simulink model "point_cloud_filter_transform_node"  (R2021b)
settings: Solver=FixedStepAuto  StartTime=0.0  StopTime=inf  RelTol=1e-3
model workspace (MAT data in the model file):
  Logfile_Data_Object = ros2bag
  Logfile_Data_Object.FilePath = 'C:\azumiken\lidars_point_raw\lidars_point_raw_0.db3'
  Logfile_Data_Object.StartTime = 1633675920681641206
  Logfile_Data_Object.EndTime = 1633676017682751873
  Logfile_Data_Object.AvailableTopics = table
  Logfile_Data_Object.AvailableTopics.data{1} = [969; 970]
  Logfile_Data_Object.AvailableTopics.data{2} = categorical
  Logfile_Data_Object.AvailableTopics.data{2}.categoryNames = {'sensor_msgs/PointCloud2'}
  Logfile_Data_Object.AvailableTopics.data{2}.codes = [1; 1]
  Logfile_Data_Object.AvailableTopics.data{3}{1} = '% contain additional information such as normals, intensity, etc. The
    | % point data is stored as a binary blob, its layout described by the
    | % contents of the "fields" array.
    | %
    | % The point cloud data may be organized 2d (image-like) or 1d (unordered).
    | % Point clouds organized as 2d images may be produced by camera depth sensors
    | % such as stereo or Time-of-flight.
    | 
    | % Time of sensor data acquisition, and the coordinate frame ID (for 3d points).
    | std_msgs/Header header
    | 
    | % 2D structure of the point cloud. If the cloud is unordered, height is
    | % 1 and width is the length of the point cloud.
    | uint32 height
    | uint32 width
    | 
    | % Describes the channels and their layout in the binary data blob.
    | PointField[] fields
    | 
    | logical    is_bigendian % Is this data bigendian?
    | uint32  point_step      % Length of a point in bytes
    | uint32  row_step        % Length of a row in bytes
    | uint8[] data            % Actual point data, size is (row_step*height)
    | 
    | logical is_dense        % True if there are no invalid points'
  Logfile_Data_Object.AvailableTopics.data{3}{2} = '% contain additional information such as normals, intensity, etc. The
    | % point data is stored as a binary blob, its layout described by the
    | % contents of the "fields" array.
    | %
    | % The point cloud data may be organized 2d (image-like) or 1d (unordered).
    | % Point clouds organized as 2d images may be produced by camera depth sensors
    | % such as stereo or Time-of-flight.
    | 
    | % Time of sensor data acquisition, and the coordinate frame ID (for 3d points).
    | std_msgs/Header header
    | 
    | % 2D structure of the point cloud. If the cloud is unordered, height is
    | % 1 and width is the length of the point cloud.
    | uint32 height
    | uint32 width
    | 
    | % Describes the channels and their layout in the binary data blob.
    | PointField[] fields
    | 
    | logical    is_bigendian % Is this data bigendian?
    | uint32  point_step      % Length of a point in bytes
    | uint32  row_step        % Length of a row in bytes
    | uint8[] data            % Actual point data, size is (row_step*height)
    | 
    | logical is_dense        % True if there are no invalid points'
  Logfile_Data_Object.AvailableTopics.ndims = 2
  Logfile_Data_Object.AvailableTopics.nrows = 2
  Logfile_Data_Object.AvailableTopics.rownames = {'/lidar_front/points_raw'; '/lidar_rear/points_raw'}
  Logfile_Data_Object.AvailableTopics.nvars = 3
  Logfile_Data_Object.AvailableTopics.varnames = {'NumMessages', 'MessageType', 'MessageDefinition'}
  Logfile_Data_Object.AvailableTopics.props.useVariableNamesOriginal = 0
  Logfile_Data_Object.AvailableTopics.props.useDimensionNamesOriginal = 0
  Logfile_Data_Object.AvailableTopics.props.CustomProps = struct()
  Logfile_Data_Object.AvailableTopics.props.VariableCustomProps = struct()
  Logfile_Data_Object.AvailableTopics.props.versionSavedFrom = 4
  Logfile_Data_Object.AvailableTopics.props.minCompatibleVersion = 1
  Logfile_Data_Object.AvailableTopics.props.incompatibilityMsg = ''
  Logfile_Data_Object.AvailableTopics.props.VersionSavedFrom = 4
  Logfile_Data_Object.AvailableTopics.props.Description = ''
  Logfile_Data_Object.AvailableTopics.props.VariableNamesOriginal = {}
  Logfile_Data_Object.AvailableTopics.props.DimensionNames = {'Row', 'Variables'}
  Logfile_Data_Object.AvailableTopics.props.DimensionNamesOriginal = {}
  Logfile_Data_Object.AvailableTopics.props.UserData = []
  Logfile_Data_Object.AvailableTopics.props.VariableDescriptions = {}
  Logfile_Data_Object.AvailableTopics.props.VariableUnits = {}
  Logfile_Data_Object.AvailableTopics.props.VariableContinuity = {}
  Logfile_Data_Object.MessageList = table
  Logfile_Data_Object.MessageList.data{1} = [1633675920681641206 1633675920704850047 1633675920710280571 1633675920841302537 1633675920849007917 1633675920944718285 1633675920950454411 1633675921046456357 1633675921051238695 1633675921143527086 1633675921154682295 1633675921262758351 ... (1939 elements, 1939x1)]
  Logfile_Data_Object.MessageList.data{2} = categorical
  Logfile_Data_Object.MessageList.data{2}.categoryNames = {'/lidar_rear/points_raw'; '/lidar_front/points_raw'}
  Logfile_Data_Object.MessageList.data{2}.codes = [1 2 1 2 1 2 1 2 1 2 1 2 ... (1939 elements, 1939x1)]
  Logfile_Data_Object.MessageList.data{3} = categorical
  Logfile_Data_Object.MessageList.data{3}.categoryNames = {'sensor_msgs/PointCloud2'}
  Logfile_Data_Object.MessageList.data{3}.codes = [1 1 1 1 1 1 1 1 1 1 1 1 ... (1939 elements, 1939x1)]
  Logfile_Data_Object.MessageList.ndims = 2
  Logfile_Data_Object.MessageList.nrows = 1939
  Logfile_Data_Object.MessageList.nvars = 3
  Logfile_Data_Object.MessageList.varnames = {'Time', 'Topic', 'MessageType'}
  Logfile_Data_Object.MessageList.props.useVariableNamesOriginal = 0
  Logfile_Data_Object.MessageList.props.useDimensionNamesOriginal = 0
  Logfile_Data_Object.MessageList.props.CustomProps = struct()
  Logfile_Data_Object.MessageList.props.VariableCustomProps = struct()
  Logfile_Data_Object.MessageList.props.versionSavedFrom = 4
  Logfile_Data_Object.MessageList.props.minCompatibleVersion = 1
  Logfile_Data_Object.MessageList.props.incompatibilityMsg = ''
  Logfile_Data_Object.MessageList.props.VersionSavedFrom = 4
  Logfile_Data_Object.MessageList.props.Description = ''
  Logfile_Data_Object.MessageList.props.VariableNamesOriginal = {}
  Logfile_Data_Object.MessageList.props.DimensionNames = {'Row', 'Variables'}
  Logfile_Data_Object.MessageList.props.DimensionNamesOriginal = {}
  Logfile_Data_Object.MessageList.props.UserData = []
  Logfile_Data_Object.MessageList.props.VariableDescriptions = {}
  Logfile_Data_Object.MessageList.props.VariableUnits = {}
  Logfile_Data_Object.MessageList.props.VariableContinuity = {}
  Logfile_Data_Object.TopicTypeMap = containers.Map
  Logfile_Data_Object.TopicTypeMap.serialization.keys = {'/lidar_front/points_raw', '/lidar_rear/points_raw'}
  Logfile_Data_Object.TopicTypeMap.serialization.values = {'sensor_msgs/PointCloud2', 'sensor_msgs/PointCloud2'}
  Logfile_Data_Object.TopicTypeMap.serialization.uniformity = 1
  Logfile_Data_Object.TopicTypeMap.serialization.keyType = 'char'
  Logfile_Data_Object.TopicTypeMap.serialization.valueType = 'char'
  Logfile_Data_Object.TopicDefinitionMap = containers.Map
  Logfile_Data_Object.TopicDefinitionMap.serialization.keys = {'/lidar_front/points_raw', '/lidar_rear/points_raw'}
  Logfile_Data_Object.TopicDefinitionMap.serialization.values{1} = '% contain additional information such as normals, intensity, etc. The
    | % point data is stored as a binary blob, its layout described by the
    | % contents of the "fields" array.
    | %
    | % The point cloud data may be organized 2d (image-like) or 1d (unordered).
    | % Point clouds organized as 2d images may be produced by camera depth sensors
    | % such as stereo or Time-of-flight.
    | 
    | % Time of sensor data acquisition, and the coordinate frame ID (for 3d points).
    | std_msgs/Header header
    | 
    | % 2D structure of the point cloud. If the cloud is unordered, height is
    | % 1 and width is the length of the point cloud.
    | uint32 height
    | uint32 width
    | 
    | % Describes the channels and their layout in the binary data blob.
    | PointField[] fields
    | 
    | logical    is_bigendian % Is this data bigendian?
    | uint32  point_step      % Length of a point in bytes
    | uint32  row_step        % Length of a row in bytes
    | uint8[] data            % Actual point data, size is (row_step*height)
    | 
    | logical is_dense        % True if there are no invalid points'
  Logfile_Data_Object.TopicDefinitionMap.serialization.values{2} = '% contain additional information such as normals, intensity, etc. The
    | % point data is stored as a binary blob, its layout described by the
    | % contents of the "fields" array.
    | %
    | % The point cloud data may be organized 2d (image-like) or 1d (unordered).
    | % Point clouds organized as 2d images may be produced by camera depth sensors
    | % such as stereo or Time-of-flight.
    | 
    | % Time of sensor data acquisition, and the coordinate frame ID (for 3d points).
    | std_msgs/Header header
    | 
    | % 2D structure of the point cloud. If the cloud is unordered, height is
    | % 1 and width is the length of the point cloud.
    | uint32 height
    | uint32 width
    | 
    | % Describes the channels and their layout in the binary data blob.
    | PointField[] fields
    | 
    | logical    is_bigendian % Is this data bigendian?
    | uint32  point_step      % Length of a point in bytes
    | uint32  row_step        % Length of a row in bytes
    | uint8[] data            % Actual point data, size is (row_step*height)
    | 
    | logical is_dense        % True if there are no invalid points'
  Logfile_Data_Object.TopicDefinitionMap.serialization.uniformity = 1
  Logfile_Data_Object.TopicDefinitionMap.serialization.keyType = 'char'
  Logfile_Data_Object.TopicDefinitionMap.serialization.valueType = 'char'
  Logfile_Path = 'C:\azumiken\lidars_point_raw\lidars_point_raw_0.db3'
  Logfile_Playback_Duration = nan
  Logfile_Playback_Offset = nan
  SL_ROS_VariableLengthArrays_MaxSizes.CommonInfo.ArrayTruncateAction = 'EmitWarning'
  SL_ROS_VariableLengthArrays_MaxSizes.MsgTypeMap = containers.Map
  SL_ROS_VariableLengthArrays_MaxSizes.MsgTypeMap.serialization.keys = {'sensor_msgs/PointCloud2'}
  SL_ROS_VariableLengthArrays_MaxSizes.MsgTypeMap.serialization.values{1}(1).PropertyName = 'data'
  SL_ROS_VariableLengthArrays_MaxSizes.MsgTypeMap.serialization.values{1}(1).DataType = 'uint8'
  SL_ROS_VariableLengthArrays_MaxSizes.MsgTypeMap.serialization.values{1}(1).MaxLength = 220000
  SL_ROS_VariableLengthArrays_MaxSizes.MsgTypeMap.serialization.values{1}(2).PropertyName = 'fields'
  SL_ROS_VariableLengthArrays_MaxSizes.MsgTypeMap.serialization.values{1}(2).DataType = 'sensor_msgs/PointField'
  SL_ROS_VariableLengthArrays_MaxSizes.MsgTypeMap.serialization.values{1}(2).MaxLength = 16
  SL_ROS_VariableLengthArrays_MaxSizes.MsgTypeMap.serialization.uniformity = 0
  SL_ROS_VariableLengthArrays_MaxSizes.MsgTypeMap.serialization.keyType = 'char'
  SL_ROS_VariableLengthArrays_MaxSizes.MsgTypeMap.serialization.valueType = 'any'
undefined symbols (not defined in the file or in its folder): height, row_step, width
libraries: ros2lib x4, simulink x4
settings Model: Creator=takum  LastModifiedBy=takumi onozawa
settings OptimizationCC: DefaultParameterBehavior=Inlined  EnhancedBackFolding=on  PassReuseOutputArgsAs=Individual arguments  ZeroExternalMemoryAtStartup=off  ZeroInternalMemoryAtStartup=off  MaxStackSize=64  OptimizeBlockOrder=speed  DifferentSizesBufferReuse=on  OptimizationCustomize=off  EfficientTunableParamExpr=on
settings DebuggingCC: ParameterTunabilityLossMsg=error
settings SFSimCC: SimParseCustomCode=off  SimTargetLang=C++
settings RTWCC: Description=Embedded Coder  SystemTargetFile=ert.tlc  HardwareBoard=Robot Operating System 2 (ROS 2)  TemplateMakefile=ert_default_tmf  Toolchain=Colcon Tools
settings CodeAppCC: ForceParamTrailComments=on  IgnoreCustomStorageClasses=off  OperatorAnnotations=on  SimulinkDataObjDesc=on  SFDataObjDesc=on  InsertBlockDesc=on
settings ERTTargetCC: TargetLangStandard=C99 (ISO)  InlinedParameterPlacement=NonHierarchical  ERTCustomFileTemplate=example_file_process.tlc

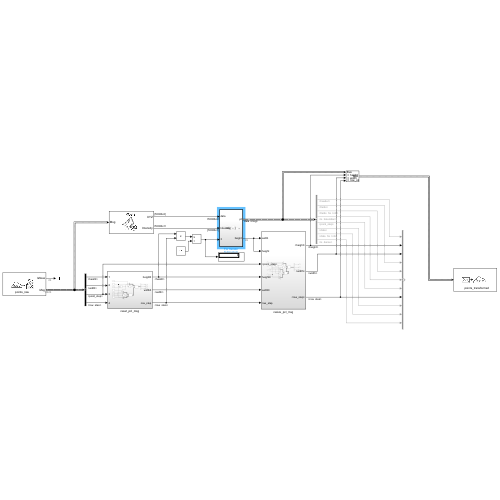
[thumbnail: Simulink's stored preview of the top-level diagram]
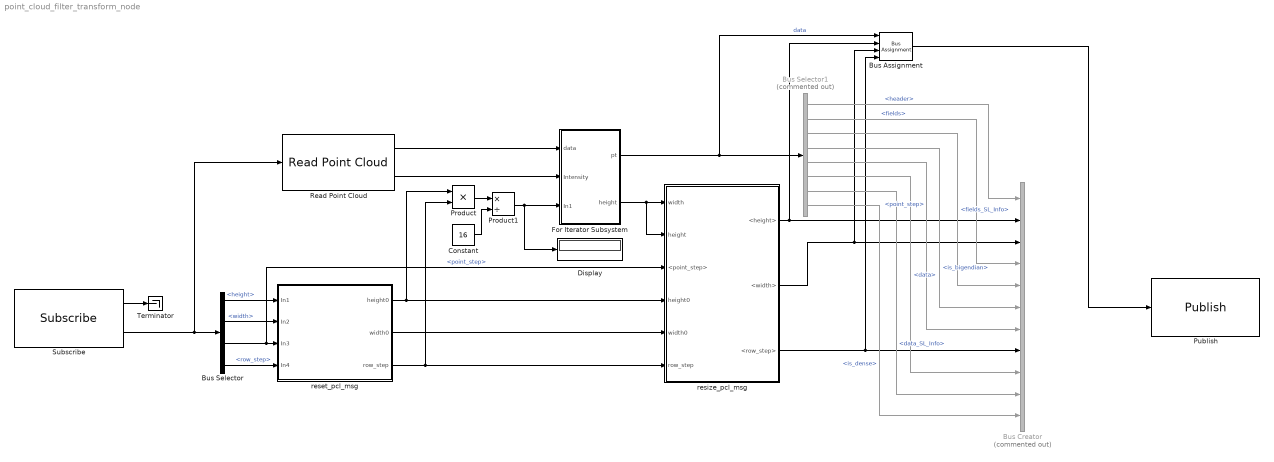
== system point_cloud_filter_transform_node ==
  Bus Assignment : BusAssignment  AssignedSignals=height,width,row_step
  Bus Creator : BusCreator  Commented=on  Inputs=11
  Bus Selector : BusSelector  OutputSignals=height,width,point_step,row_step
  Bus Selector1 : BusSelector  Commented=on  OutputSignals=header,fields,fields_SL_Info,is_bigendian,point_step,data,data_SL_Info,is_dense
  Constant : Constant  Value=16  OutDataTypeStr=uint32
  Display : Display
  For Iterator Subsystem : Subsystem  TreatAsAtomicUnit=on
  Product : Product  OutDataTypeStr=uint32
  Product1 : Product  Inputs=*/  OutDataTypeStr=uint32
  Publish : ros2lib/Publish  topicSource=Specify your own  topic=points_transformed  messageType=sensor_msgs/PointCloud2  QOSHistory=Keep last  QOSDepth=1  QOSReliability=Reliable  QOSDurability=Volatile
      settings: SourceProductBaseCode=RR
  Read Point Cloud : ros2lib/Read Point Cloud  MaximumPointCloudSize=[1, 55000]  PreserveStructure=off  ShowRGBOutput=off  ShowIntensityOutput=on  ShowErrorCodeOutput=off  VariableSizeOutputs=off
      settings: SourceProductBaseCode=RR
  Subscribe : ros2lib/Subscribe  topicSource=Specify your own  topic=points_raw  messageType=sensor_msgs/PointCloud2  sampleTime=-1  QOSHistory=Keep last  QOSDepth=1  QOSReliability=Reliable  QOSDurability=Volatile
      settings: SourceProductBaseCode=RR
  Terminator : Terminator
  reset_pcl_msg : Subsystem
  resize_pcl_msg : Subsystem
  wires:
  Subscribe/1 -> Terminator/1
  Bus Assignment/1 -> Publish/1
  resize_pcl_msg/1(<height>) -> Bus Assignment/2, Bus Creator/2
  Subscribe/2 -> Bus Selector/1, Read Point Cloud/1
  Bus Selector/2 -> reset_pcl_msg/2(In2)  "<width>"
  reset_pcl_msg/1(height0) -> resize_pcl_msg/4(height0), Product/1
  Product/1 -> Product1/1
  Bus Selector/4 -> reset_pcl_msg/4(In4)  "<row_step>"
  Product1/1 -> Display/1, For Iterator Subsystem/3(In1)
  For Iterator Subsystem/2(height) -> resize_pcl_msg/2(height), resize_pcl_msg/1(width)
  reset_pcl_msg/2(width0) -> resize_pcl_msg/5(width0)
  Constant/1 -> Product1/2
  reset_pcl_msg/3(row_step) -> resize_pcl_msg/6(row_step), Product/2
  Bus Selector/1 -> reset_pcl_msg/1(In1)  "<height>"
  Bus Selector/3 -> resize_pcl_msg/3(<point_step>), reset_pcl_msg/3(In3)  "<point_step>"
  resize_pcl_msg/3(<row_step>) -> Bus Assignment/4, Bus Creator/8
  resize_pcl_msg/2(<width>) -> Bus Assignment/3, Bus Creator/3
  Read Point Cloud/1 -> For Iterator Subsystem/1(data)
  Read Point Cloud/2 -> For Iterator Subsystem/2(Intensity)
  For Iterator Subsystem/1(pt) -> Bus Assignment/1, Bus Selector1/1  "data"
  Bus Selector1/1 -> Bus Creator/1  "<header>"
  Bus Selector1/2 -> Bus Creator/4  "<fields>"
  Bus Selector1/3 -> Bus Creator/5  "<fields_SL_Info>"
  Bus Selector1/4 -> Bus Creator/6  "<is_bigendian>"
  Bus Selector1/5 -> Bus Creator/7  "<point_step>"
  Bus Selector1/6 -> Bus Creator/9  "<data>"
  Bus Selector1/7 -> Bus Creator/10  "<data_SL_Info>"
  Bus Selector1/8 -> Bus Creator/11  "<is_dense>"

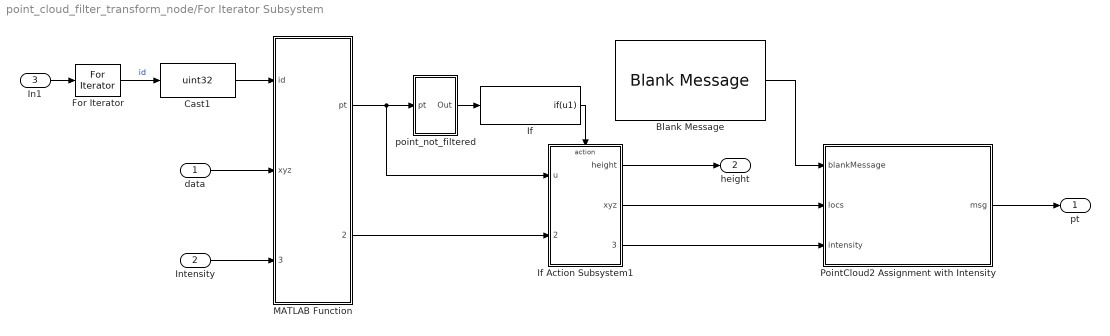
== system point_cloud_filter_transform_node/For Iterator Subsystem ==
  data : Inport
  Intensity : Inport  Port=2
  In1 : Inport  Port=3
  Blank Message : ros2lib/Blank Message  messageClass=Message  entityType=sensor_msgs/PointCloud2  messageType=sensor_msgs/PointCloud2  SampleTime=inf
      settings: SourceProductBaseCode=RR
  Cast1 : DataTypeConversion  OutDataTypeStr=uint32
  For Iterator : ForIterator  IterationSource=external
  If : If  IfExpression=u1  ShowElse=off
  If Action Subsystem1 : Subsystem  TreatAsAtomicUnit=on
  MATLAB Function : MATLAB Function  TreatAsAtomicUnit=on
  PointCloud2 Assignment with Intensity : MATLAB Function  TreatAsAtomicUnit=on
  point_not_filtered : Subsystem
  pt : Outport
  height : Outport  Port=2
  wires:
  If Action Subsystem1/2(xyz) -> PointCloud2 Assignment with Intensity/2(locs)
  If Action Subsystem1/3(intensity) -> PointCloud2 Assignment with Intensity/3(intensity)
  If Action Subsystem1/1(height) -> height/1
  Cast1/1 -> MATLAB Function/1(id)
  PointCloud2 Assignment with Intensity/1(msg) -> pt/1
  Intensity/1 -> MATLAB Function/3(Intensity)
  For Iterator/1 -> Cast1/1  "id"
  data/1 -> MATLAB Function/2(xyz)
  MATLAB Function/1(pt) -> If Action Subsystem1/1(u), point_not_filtered/1(pt)
  point_not_filtered/1(Out) -> If/1
  In1/1 -> For Iterator/1
  Blank Message/1 -> PointCloud2 Assignment with Intensity/1(blankMessage)
  MATLAB Function/2(intensity) -> If Action Subsystem1/2(Intensity)
  If/1 -> If Action Subsystem1/Action

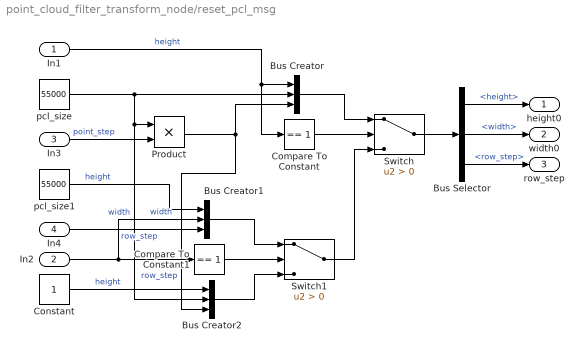
== system point_cloud_filter_transform_node/reset_pcl_msg ==
  In1 : Inport
  In2 : Inport  Port=2
  In3 : Inport  Port=3
  In4 : Inport  Port=4
  Bus Creator : BusCreator  Inputs=3
  Bus Creator1 : BusCreator  Inputs=3
  Bus Creator2 : BusCreator  Inputs=3
  Bus Selector : BusSelector  OutputSignals=height,width,row_step
  Compare To Constant : simulink/Logic and Bit Operations/Compare To Constant  relop===  const=1  OutDataTypeStr=boolean
  Compare To Constant1 : simulink/Logic and Bit Operations/Compare To Constant  relop===  const=1  OutDataTypeStr=boolean
  Constant : Constant  OutDataTypeStr=uint32
  Product : Product  OutDataTypeStr=uint32
  Switch : Switch  Criteria=u2 > Threshold
  Switch1 : Switch  Criteria=u2 > Threshold
  pcl_size : Constant  Value=55000  OutDataTypeStr=uint32
  pcl_size1 : Constant  Value=55000  OutDataTypeStr=uint32
  height0 : Outport
  width0 : Outport  Port=2
  row_step : Outport  Port=3
  wires:
  In3/1 -> Product/2  "point_step"
  In1/1 -> Compare To Constant/1, Bus Creator/1  "height"
  Compare To Constant/1 -> Switch/2
  Bus Creator/1 -> Switch/1
  Compare To Constant1/1 -> Switch1/2
  pcl_size1/1 -> Bus Creator1/1  "height"
  Bus Creator1/1 -> Switch1/1
  In2/1 -> Bus Creator1/2, Compare To Constant1/1  "width"
  In4/1 -> Bus Creator1/3  "row_step"
  Switch1/1 -> Switch/3
  Product/1 -> Bus Creator2/3, Bus Creator/3  "row_step"
  pcl_size/1 -> Bus Creator/2, Bus Creator2/2, Product/1  "width"
  Constant/1 -> Bus Creator2/1  "height"
  Bus Creator2/1 -> Switch1/3
  Switch/1 -> Bus Selector/1
  Bus Selector/2 -> width0/1  "<width>"
  Bus Selector/1 -> height0/1  "<height>"
  Bus Selector/3 -> row_step/1  "<row_step>"

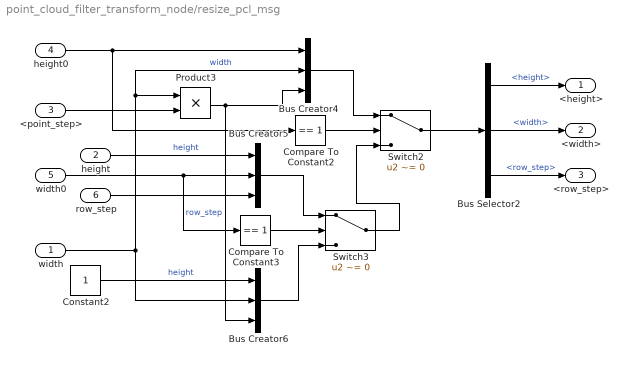
== system point_cloud_filter_transform_node/resize_pcl_msg ==
  width : Inport
  height : Inport  Port=2
  <point_step> : Inport  Port=3
  height0 : Inport  Port=4
  width0 : Inport  Port=5
  row_step : Inport  Port=6
  Bus Creator4 : BusCreator  Inputs=3
  Bus Creator5 : BusCreator  Inputs=3
  Bus Creator6 : BusCreator  Inputs=3
  Bus Selector2 : BusSelector  OutputSignals=height,width,row_step
  Compare To Constant2 : simulink/Logic and Bit Operations/Compare To Constant  relop===  const=1  OutDataTypeStr=boolean
  Compare To Constant3 : simulink/Logic and Bit Operations/Compare To Constant  relop===  const=1  OutDataTypeStr=boolean
  Constant2 : Constant  OutDataTypeStr=uint32
  Product3 : Product  OutDataTypeStr=uint32
  Switch2 : Switch  Criteria=u2 ~= 0
  Switch3 : Switch  Criteria=u2 ~= 0
  <height> : Outport
  <width> : Outport  Port=2
  <row_step> : Outport  Port=3
  wires:
  Compare To Constant3/1 -> Switch3/2
  Bus Creator6/1 -> Switch3/3
  Switch2/1 -> Bus Selector2/1
  Product3/1 -> Bus Creator4/3, Bus Creator6/3  "row_step"
  Switch3/1 -> Switch2/3
  Bus Selector2/1 -> <height>/1  "<height>"
  width/1 -> Bus Creator6/2, Bus Creator4/2, Product3/1  "width"
  Bus Creator5/1 -> Switch3/1
  Constant2/1 -> Bus Creator6/1  "height"
  Bus Creator4/1 -> Switch2/1
  Compare To Constant2/1 -> Switch2/2
  height0/1 -> Compare To Constant2/1, Bus Creator4/1
  width0/1 -> Compare To Constant3/1, Bus Creator5/2
  Bus Selector2/3 -> <row_step>/1  "<row_step>"
  <point_step>/1 -> Product3/2
  row_step/1 -> Bus Creator5/3
  Bus Selector2/2 -> <width>/1  "<width>"
  height/1 -> Bus Creator5/1  "height"

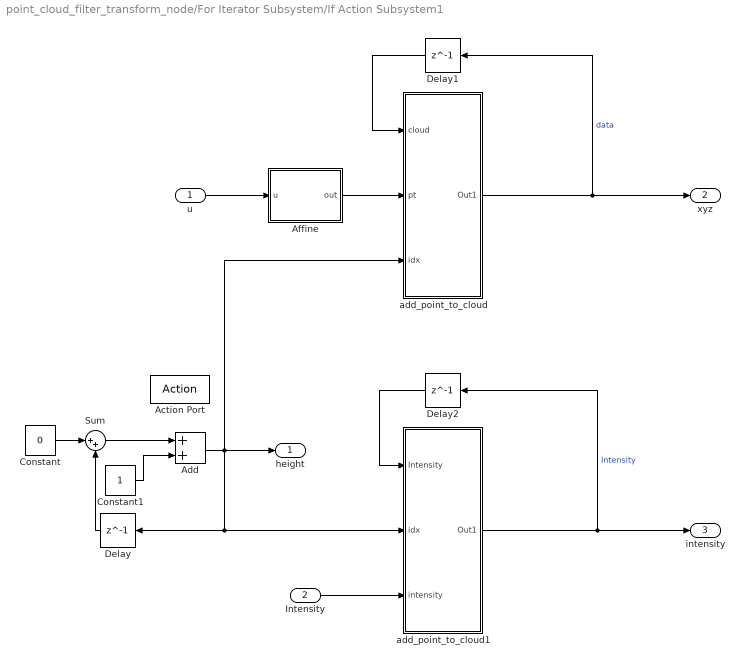
== system point_cloud_filter_transform_node/For Iterator Subsystem/If Action Subsystem1 ==
  u : Inport
  Intensity : Inport  Port=2
  Action Port : ActionPort  ActionPortLabel=if(u1)
  Add : Sum
  Affine : MATLAB Function  TreatAsAtomicUnit=on
  Constant : Constant  Value=0
  Constant1 : Constant
  Delay : Delay  DelayLength=1
  Delay1 : Delay  DelayLength=1  InitialCondition=0
  Delay2 : Delay  DelayLength=1  InitialCondition=0
  Sum : Sum  Inputs=|++
  add_point_to_cloud : Subsystem
  add_point_to_cloud1 : Subsystem
  height : Outport
  xyz : Outport  Port=2
  intensity : Outport  Port=3
  wires:
  u/1 -> Affine/1(u)
  Delay1/1 -> add_point_to_cloud/1(cloud)
  Add/1 -> add_point_to_cloud/3(idx), Delay/1, add_point_to_cloud1/2(idx), height/1
  Constant1/1 -> Add/2
  Sum/1 -> Add/1
  Constant/1 -> Sum/1
  Delay/1 -> Sum/2
  add_point_to_cloud/1(Out1) -> xyz/1, Delay1/1  "data"
  Affine/1(out) -> add_point_to_cloud/2(pt)
  Intensity/1 -> add_point_to_cloud1/3(intensity)
  Delay2/1 -> add_point_to_cloud1/1(Intensity)
  add_point_to_cloud1/1(Out1) -> Delay2/1, intensity/1  "Intensity"

== system point_cloud_filter_transform_node/For Iterator Subsystem/point_not_filtered ==
  pt : Inport
  Logical Operator2 : Logic  AllPortsSameDT=off  OutDataTypeStr=boolean
  m_angle_filter : Subsystem
  m_distance_filter : Subsystem
  Out : Outport
  wires:
  pt/1 -> m_angle_filter/1(pt), m_distance_filter/1(pt)
  Logical Operator2/1 -> Out/1
  m_distance_filter/1(Out1) -> Logical Operator2/2
  m_angle_filter/1(Out1) -> Logical Operator2/1

== system point_cloud_filter_transform_node/For Iterator Subsystem/If Action Subsystem1/add_point_to_cloud ==
  cloud : Inport
  pt : Inport  Port=2
  idx : Inport  Port=3
  MATLAB Function : MATLAB Function  TreatAsAtomicUnit=on
  MATLAB Function1 : MATLAB Function  TreatAsAtomicUnit=on
  Switch : Switch  Criteria=u2 ~= 0
  Out1 : Outport
  wires:
  MATLAB Function/1(cloud) -> Switch/1
  cloud/1 -> Switch/2, MATLAB Function/1("cloud ")
  pt/1 -> MATLAB Function1/1(pt), MATLAB Function/2(pt)
  idx/1 -> MATLAB Function/3(idx)
  Switch/1 -> Out1/1
  MATLAB Function1/1(cloud) -> Switch/3

== system point_cloud_filter_transform_node/For Iterator Subsystem/If Action Subsystem1/add_point_to_cloud1 ==
  Intensity : Inport
  idx : Inport  Port=2
  intensity : Inport  Port=3
  MATLAB Function : MATLAB Function  TreatAsAtomicUnit=on
  MATLAB Function2 : MATLAB Function  TreatAsAtomicUnit=on
  Switch : Switch  Criteria=u2 ~= 0
  Out1 : Outport
  wires:
  idx/1 -> MATLAB Function/2(j)
  intensity/1 -> MATLAB Function2/1(intensity), MATLAB Function/3(intensity)
  Intensity/1 -> MATLAB Function/1("Intensity "), Switch/2
  MATLAB Function2/1(Intensity) -> Switch/3
  MATLAB Function/1(Intensity) -> Switch/1
  Switch/1 -> Out1/1

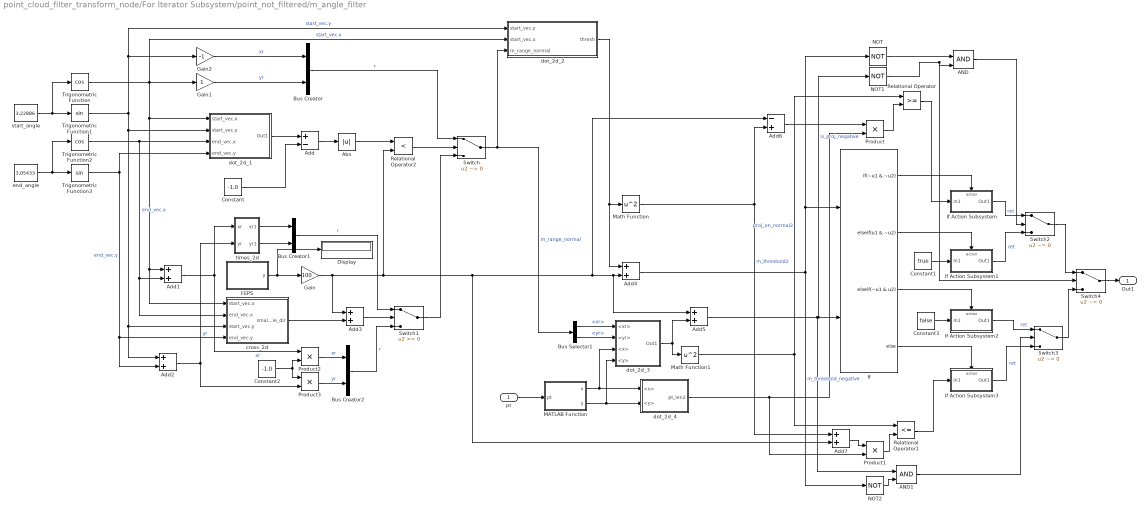
== system point_cloud_filter_transform_node/For Iterator Subsystem/point_not_filtered/m_angle_filter ==
  pt : Inport
  AND : Logic  IconShape=distinctive  AllPortsSameDT=off  OutDataTypeStr=boolean
  AND1 : Logic  IconShape=distinctive  AllPortsSameDT=off  OutDataTypeStr=boolean
  Abs : Abs
  Add : Sum  Inputs=+-
  Add{1..5,7} (6 alike) : Sum
  Add6 : Sum  Inputs=-+
  Bus Creator : BusCreator  Inputs=2
  Bus Creator1 : BusCreator  Inputs=2
  Bus Creator2 : BusCreator  Inputs=2
  Bus Selector1 : BusSelector  OutputSignals=xr,yr
  Constant : Constant  Value=-1.0
  Constant1 : Constant  Value=true  OutDataTypeStr=boolean
  Constant2 : Constant  Value=-1.0
  Constant3 : Constant  Value=false  OutDataTypeStr=boolean
  Display : Display
  FEPS : MATLAB Function  TreatAsAtomicUnit=on
  Gain : Gain  Gain=100
  Gain1 : Gain
  Gain2 : Gain  Gain=-1
  If : If  NumInputs=2  IfExpression=~u1 & ~u2  ElseIfExpressions=u1 & ~u2, ~u1 & u2
  If Action Subsystem : Subsystem  TreatAsAtomicUnit=on
  If Action Subsystem1 : Subsystem  TreatAsAtomicUnit=on
  If Action Subsystem2 : Subsystem  TreatAsAtomicUnit=on
  If Action Subsystem3 : Subsystem  TreatAsAtomicUnit=on
  MATLAB Function : MATLAB Function  TreatAsAtomicUnit=on
  Math Function : Math  Operator=square  SaturateOnIntegerOverflow=on
  Math Function1 : Math  Operator=square  SaturateOnIntegerOverflow=on
  NOT : Logic  Operator=NOT  IconShape=distinctive  AllPortsSameDT=off  OutDataTypeStr=boolean
  NOT1 : Logic  Operator=NOT  IconShape=distinctive  AllPortsSameDT=off  OutDataTypeStr=boolean
  NOT2 : Logic  Operator=NOT  IconShape=distinctive  AllPortsSameDT=off  OutDataTypeStr=boolean
  Product{,1..3} (4 alike) : Product
  Relational Operator : RelationalOperator  OutDataTypeStr=boolean  RndMeth=Simplest
  Relational Operator1 : RelationalOperator  Operator=<=  OutDataTypeStr=boolean  RndMeth=Simplest
  Relational Operator2 : RelationalOperator  Operator=<  OutDataTypeStr=boolean  RndMeth=Simplest
  Switch{,2..4} (4 alike) : Switch  Criteria=u2 ~= 0
  Switch1 : Switch
  Trigonometric Function : Trigonometry  Operator=cos
  Trigonometric Function1 : Trigonometry
  Trigonometric Function2 : Trigonometry  Operator=cos
  Trigonometric Function3 : Trigonometry
  cross_2d : Subsystem
  dot_2d_1 : Subsystem
  dot_2d_2 : Subsystem
  dot_2d_3 : Subsystem
  dot_2d_4 : Subsystem
  end_angle : Constant  Value=3.05433
  start_angle : Constant  Value=3.22886
  times_2d : Subsystem
  Out1 : Outport
  wires:
  pt/1 -> MATLAB Function/1(pt)
  start_angle/1 -> Trigonometric Function1/1, Trigonometric Function/1
  end_angle/1 -> Trigonometric Function3/1, Trigonometric Function2/1
  Trigonometric Function/1 -> dot_2d_2/2(start_vec.x), cross_2d/1(start_vec.x), Add1/1, dot_2d_1/1(start_vec.x), Gain1/1  "start_vec.x"
  Trigonometric Function1/1 -> dot_2d_1/2(start_vec.y), Add2/1, cross_2d/3(start_vec.y), dot_2d_2/1(start_vec.y), Gain2/1  "start_vec.y"
  Trigonometric Function2/1 -> cross_2d/2(end_vec.x), Add1/2, dot_2d_1/3(end_vec.x)  "end_vec.x"
  Trigonometric Function3/1 -> Add2/2, cross_2d/4(end_vec.y), dot_2d_1/4(end_vec.y)  "end_vec.y"
  dot_2d_1/1(Out1) -> Add/1
  Constant/1 -> Add/2
  Add/1 -> Abs/1
  FEPS/1(y) -> Gain/1, Display/1
  Abs/1 -> Relational Operator2/1
  Relational Operator2/1 -> Switch/2
  Gain1/1 -> Bus Creator/2  "yr"
  Gain2/1 -> Bus Creator/1  "xr"
  Bus Creator/1 -> Switch/1  "r"
  Add1/1 -> times_2d/1(xr), Product2/1  "xr"
  Add2/1 -> times_2d/2(yr), Product3/2  "yr"
  Switch1/1 -> Switch/3
  Product3/1 -> Bus Creator2/2  "yr"
  Bus Creator2/1 -> Switch1/3  "r"
  Product2/1 -> Bus Creator2/1  "xr"
  Bus Creator1/1 -> Switch1/1  "r"
  Constant2/1 -> Product2/2, Product3/1
  Add3/1 -> Switch1/2
  cross_2d/1(small_angle_dir) -> Add3/2
  times_2d/1(xr1) -> Bus Creator1/1
  times_2d/2(yr1) -> Bus Creator1/2
  Switch/1 -> Bus Selector1/1, dot_2d_2/3(m_range_normal)  "m_range_normal"
  dot_2d_2/1(thresh) -> Add4/1, Math Function/1
  Math Function/1 -> Add6/2, Add7/1  "m_threshold2"
  Add4/1 -> NOT2/1, NOT/1, If/1  "m_threshold_negative"
  Gain/1 -> Add3/1, Relational Operator2/2, Add7/2, Add6/1, Add5/1, Add4/2
  Math Function1/1 -> Relational Operator1/1, Relational Operator/1  "proj_on_normal2"
  Add5/1 -> AND1/1, NOT1/1, If/2  "is_proj_negative"
  If/1 -> If Action Subsystem/Action
  If/2 -> If Action Subsystem1/Action
  If/3 -> If Action Subsystem2/Action
  If/4 -> If Action Subsystem3/Action
  Constant3/1 -> If Action Subsystem2/1(In1)
  Constant1/1 -> If Action Subsystem1/1(In1)
  If Action Subsystem1/1(Out1) -> Switch2/3  "ret"
  If Action Subsystem2/1(Out1) -> Switch3/1  "ret"
  If Action Subsystem/1(Out1) -> Switch2/1  "ret"
  If Action Subsystem3/1(Out1) -> Switch3/3  "ret"
  AND/1 -> Switch2/2
  NOT/1 -> AND/1
  NOT1/1 -> AND/2, Switch4/2
  NOT2/1 -> AND1/2
  AND1/1 -> Switch3/2
  Switch2/1 -> Switch4/1
  Switch3/1 -> Switch4/3
  Add6/1 -> Product/1
  Product/1 -> Relational Operator/2
  Add7/1 -> Product1/1
  Product1/1 -> Relational Operator1/2
  Relational Operator/1 -> If Action Subsystem/1(In1)
  Relational Operator1/1 -> If Action Subsystem3/1(In1)
  Switch4/1 -> Out1/1
  MATLAB Function/1(x) -> dot_2d_3/3(<x>), dot_2d_4/1(<x>)
  MATLAB Function/2(y) -> dot_2d_3/4(<y>), dot_2d_4/2(<y>)
  dot_2d_4/1(pt_len2) -> Product/2, Product1/2
  dot_2d_3/1(Out1) -> Math Function1/1, Add5/2
  Bus Selector1/1 -> dot_2d_3/1(<xr>)  "<xr>"
  Bus Selector1/2 -> dot_2d_3/2(<yr>)  "<yr>"

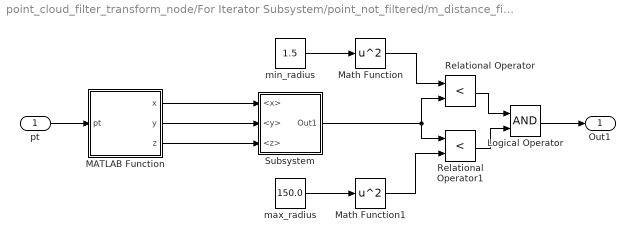
== system point_cloud_filter_transform_node/For Iterator Subsystem/point_not_filtered/m_distance_filter ==
  pt : Inport
  Logical Operator : Logic  AllPortsSameDT=off  OutDataTypeStr=boolean
  MATLAB Function : MATLAB Function  TreatAsAtomicUnit=on
  Math Function : Math  Operator=square  SaturateOnIntegerOverflow=on
  Math Function1 : Math  Operator=square  SaturateOnIntegerOverflow=on
  Relational Operator : RelationalOperator  Operator=<  OutDataTypeStr=boolean  RndMeth=Simplest
  Relational Operator1 : RelationalOperator  Operator=<  OutDataTypeStr=boolean  RndMeth=Simplest
  Subsystem : Subsystem
  max_radius : Constant  Value=150.0
  min_radius : Constant  Value=1.5
  Out1 : Outport
  wires:
  max_radius/1 -> Math Function1/1
  pt/1 -> MATLAB Function/1(pt)
  Relational Operator1/1 -> Logical Operator/2
  Relational Operator/1 -> Logical Operator/1
  min_radius/1 -> Math Function/1
  Logical Operator/1 -> Out1/1
  Math Function/1 -> Relational Operator/1
  Math Function1/1 -> Relational Operator1/2
  Subsystem/1(Out1) -> Relational Operator1/1, Relational Operator/2
  MATLAB Function/1(x) -> Subsystem/1(<x>)
  MATLAB Function/2(y) -> Subsystem/2(<y>)
  MATLAB Function/3(z) -> Subsystem/3(<z>)

== system point_cloud_filter_transform_node/For Iterator Subsystem/point_not_filtered/m_angle_filter/If Action Subsystem ==
  In1 : Inport
  Action Port : ActionPort  ActionPortLabel=if(~u1 & ~u2)
  Out1 : Outport
  wires:
  In1/1 -> Out1/1

== system point_cloud_filter_transform_node/For Iterator Subsystem/point_not_filtered/m_angle_filter/If Action Subsystem1 ==
  In1 : Inport
  Action Port : ActionPort  ActionPortLabel=elseif(u1 & ~u2)
  Out1 : Outport
  wires:
  In1/1 -> Out1/1

== system point_cloud_filter_transform_node/For Iterator Subsystem/point_not_filtered/m_angle_filter/If Action Subsystem2 ==
  In1 : Inport
  Action Port : ActionPort  ActionPortLabel=elseif( ~u1 & u2)
  Out1 : Outport
  wires:
  In1/1 -> Out1/1

== system point_cloud_filter_transform_node/For Iterator Subsystem/point_not_filtered/m_angle_filter/If Action Subsystem3 ==
  In1 : Inport
  Action Port : ActionPort  ActionPortLabel=else
  Out1 : Outport
  wires:
  In1/1 -> Out1/1

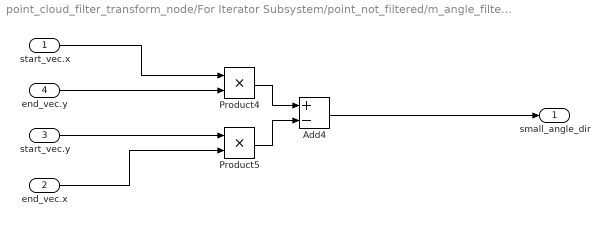
== system point_cloud_filter_transform_node/For Iterator Subsystem/point_not_filtered/m_angle_filter/cross_2d ==
  start_vec.x : Inport
  end_vec.x : Inport  Port=2
  start_vec.y : Inport  Port=3
  end_vec.y : Inport  Port=4
  Add4 : Sum  Inputs=+-
  Product4 : Product
  Product5 : Product
  small_angle_dir : Outport
  wires:
  end_vec.y/1 -> Product4/2
  Product5/1 -> Add4/2
  Product4/1 -> Add4/1
  start_vec.y/1 -> Product5/1
  Add4/1 -> small_angle_dir/1
  start_vec.x/1 -> Product4/1
  end_vec.x/1 -> Product5/2

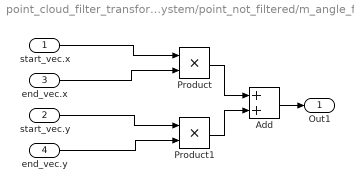
== system point_cloud_filter_transform_node/For Iterator Subsystem/point_not_filtered/m_angle_filter/dot_2d_1 ==
  start_vec.x : Inport
  start_vec.y : Inport  Port=2
  end_vec.x : Inport  Port=3
  end_vec.y : Inport  Port=4
  Add : Sum
  Product : Product
  Product1 : Product
  Out1 : Outport
  wires:
  Product/1 -> Add/1
  Product1/1 -> Add/2
  Add/1 -> Out1/1
  start_vec.y/1 -> Product1/1
  end_vec.x/1 -> Product/2
  end_vec.y/1 -> Product1/2
  start_vec.x/1 -> Product/1

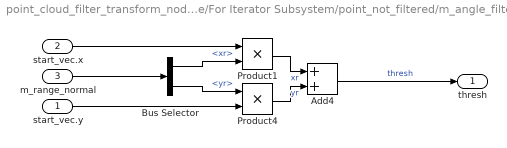
== system point_cloud_filter_transform_node/For Iterator Subsystem/point_not_filtered/m_angle_filter/dot_2d_2 ==
  start_vec.y : Inport
  start_vec.x : Inport  Port=2
  m_range_normal : Inport  Port=3
  Add4 : Sum
  Bus Selector : BusSelector  OutputSignals=xr,yr
  Product1 : Product
  Product4 : Product
  thresh : Outport
  wires:
  m_range_normal/1 -> Bus Selector/1
  Bus Selector/1 -> Product1/2  "<xr>"
  Bus Selector/2 -> Product4/1  "<yr>"
  Product1/1 -> Add4/1  "xr"
  start_vec.y/1 -> Product4/2
  Product4/1 -> Add4/2  "yr"
  start_vec.x/1 -> Product1/1
  Add4/1 -> thresh/1  "thresh"

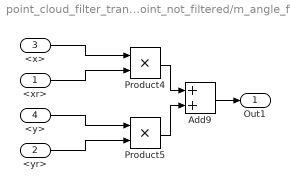
== system point_cloud_filter_transform_node/For Iterator Subsystem/point_not_filtered/m_angle_filter/dot_2d_3 ==
  <xr> : Inport
  <yr> : Inport  Port=2
  <x> : Inport  Port=3
  <y> : Inport  Port=4
  Add9 : Sum
  Product4 : Product
  Product5 : Product
  Out1 : Outport
  wires:
  Product5/1 -> Add9/2
  <x>/1 -> Product4/1
  <y>/1 -> Product5/1
  Product4/1 -> Add9/1
  <xr>/1 -> Product4/2
  Add9/1 -> Out1/1
  <yr>/1 -> Product5/2

== system point_cloud_filter_transform_node/For Iterator Subsystem/point_not_filtered/m_angle_filter/dot_2d_4 ==
  <x> : Inport
  <y> : Inport  Port=2
  Add8 : Sum
  Math Function2 : Math  Operator=square  SaturateOnIntegerOverflow=on
  Math Function3 : Math  Operator=square  SaturateOnIntegerOverflow=on
  pt_len2 : Outport
  wires:
  <y>/1 -> Math Function3/1
  Math Function3/1 -> Add8/2
  Math Function2/1 -> Add8/1
  Add8/1 -> pt_len2/1  "pt_len2"
  <x>/1 -> Math Function2/1

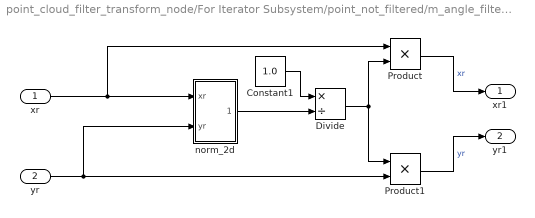
== system point_cloud_filter_transform_node/For Iterator Subsystem/point_not_filtered/m_angle_filter/times_2d ==
  xr : Inport
  yr : Inport  Port=2
  Constant1 : Constant  Value=1.0
  Divide : Product  Inputs=*/
  Product : Product
  Product1 : Product
  norm_2d : Subsystem
  xr1 : Outport
  yr1 : Outport  Port=2
  wires:
  Constant1/1 -> Divide/1
  norm_2d/1(Out1) -> Divide/2
  Product/1 -> xr1/1  "xr"
  Divide/1 -> Product1/1, Product/2
  xr/1 -> norm_2d/1(xr), Product/1
  Product1/1 -> yr1/1  "yr"
  yr/1 -> Product1/2, norm_2d/2(yr)

== system point_cloud_filter_transform_node/For Iterator Subsystem/point_not_filtered/m_distance_filter/Subsystem ==
  <x> : Inport
  <y> : Inport  Port=2
  <z> : Inport  Port=3
  Add : Sum  Inputs=3
  Math Function2 : Math  Operator=square  SaturateOnIntegerOverflow=on
  Math Function3 : Math  Operator=square  SaturateOnIntegerOverflow=on
  Math Function4 : Math  Operator=square  SaturateOnIntegerOverflow=on
  Out1 : Outport
  wires:
  <z>/1 -> Math Function4/1
  Math Function4/1 -> Add/3
  <y>/1 -> Math Function3/1
  Math Function2/1 -> Add/1
  Math Function3/1 -> Add/2
  Add/1 -> Out1/1
  <x>/1 -> Math Function2/1

== system point_cloud_filter_transform_node/For Iterator Subsystem/point_not_filtered/m_angle_filter/times_2d/norm_2d ==
  xr : Inport
  yr : Inport  Port=2
  Sqrt : Sqrt  SaturateOnIntegerOverflow=on
  dot_2d : Subsystem
  Out1 : Outport
  wires:
  Sqrt/1 -> Out1/1
  xr/1 -> dot_2d/1(In1)
  yr/1 -> dot_2d/2(In2)
  dot_2d/1(Out1) -> Sqrt/1

== system point_cloud_filter_transform_node/For Iterator Subsystem/point_not_filtered/m_angle_filter/times_2d/norm_2d/dot_2d ==
  In1 : Inport
  In2 : Inport  Port=2
  Add3 : Sum
  Math Function : Math  Operator=square  SaturateOnIntegerOverflow=on
  Math Function1 : Math  Operator=square  SaturateOnIntegerOverflow=on
  Out1 : Outport
  wires:
  Math Function/1 -> Add3/1
  Math Function1/1 -> Add3/2
  In2/1 -> Math Function1/1
  Add3/1 -> Out1/1
  In1/1 -> Math Function/1

== matlab function point_cloud_filter_transform_node/For Iterator Subsystem/MATLAB Function ==
  data: pt output; id input; xyz input; Intensity input; intensity output
function [pt,intensity] = fcn(id, xyz, Intensity)

pt = xyz(id,:);
intensity = Intensity(id);

== matlab function point_cloud_filter_transform_node/For Iterator Subsystem/If Action Subsystem1/add_point_to_cloud/MATLAB Function1 ==
  data: cloud output; pt input
function cloud = fcn(pt)
cloud = zeros(55000,3);
cloud(1,:) = pt;

== matlab function point_cloud_filter_transform_node/For Iterator Subsystem/point_not_filtered/m_angle_filter/FEPS ==
  data: y output
function y = fcn()

y = eps();

== matlab function point_cloud_filter_transform_node/For Iterator Subsystem/point_not_filtered/m_angle_filter/MATLAB Function ==
  data: x output; pt input; y output
function [x,y] = fcn(pt)
x = pt(1,1);
y = pt(1,2);

== matlab function point_cloud_filter_transform_node/For Iterator Subsystem/point_not_filtered/m_distance_filter/MATLAB Function ==
  data: x output; pt input; y output; z output
function [x,y,z] = fcn(pt)
x = pt(1,1);
y = pt(1,2);
z = pt(1,3);

== matlab function point_cloud_filter_transform_node/For Iterator Subsystem/If Action Subsystem1/add_point_to_cloud1/MATLAB Function2 ==
  data: Intensity output; intensity input
function Intensity = fcn(intensity)
Intensity = zeros(55000,1);
Intensity(1,:) = intensity;

== matlab function point_cloud_filter_transform_node/For Iterator Subsystem/PointCloud2 Assignment with Intensity ==
  data: blankMessage input Bus: SL_Bus_sensor_msgs_PointCloud2; locs input; msg output Bus: SL_Bus_sensor_msgs_PointCloud2; intensity input
function msg = assignNestedArrayMessages(blankMessage,locs,intensity)
%#codegen

blankMessage.header.frame_id(1:3) = uint8('map');
blankMessage.header.frame_id_SL_Info.CurrentLength = uint32(3);
blankMessage.height = uint32(1);
blankMessage.width = uint32(size(locs,1));
blankMessage.point_step = uint32(32);
blankMessage.row_step = blankMessage.width * blankMessage.point_step;
blankMessage.fields_SL_Info.CurrentLength = uint32(4);
blankMessage.fields(1).name(1) = uint8('x');
blankMessage.fields(1).name_SL_Info.CurrentLength = uint32(1);
blankMessage.fields(1).offset = uint32(0);
blankMessage.fields(1).datatype = uint8(7);
blankMessage.fields(1).count = uint32(1);
blankMessage.fields(2).name(1) = uint8('y');
blankMessage.fields(2).name_SL_Info.CurrentLength = uint32(1);
blankMessage.fields(2).offset = uint32(4);
blankMessage.fields(2).datatype = uint8(7);
blankMessage.fields(2).count = uint32(1);
blankMessage.fields(3).name(1) = uint8('z');
blankMessage.fields(3).name_SL_Info.CurrentLength = uint32(1);
blankMessage.fields(3).offset = uint32(8);
blankMessage.fields(3).datatype = uint8(7);
blankMessage.fields(3).count = uint32(1);
blankMessage.fields(4).name(1:9) = uint8('intensity');
blankMessage.fields(4).name_SL_Info.CurrentLength = uint32(9);
blankMessage.fields(4).offset = uint32(16);
blankMessage.fields(4).datatype = uint8(7);
blankMessage.fields(4).count = uint32(1);

locs = reshape(locs,[],3);
intensity = reshape(intensity,[],1);
data = [locs zeros(size(locs,1),1,'single') intensity zeros(size(locs,1),3,'single')];
dataPacked = reshape(permute(data,[2 1]),[],1);
dataCasted = typecast(dataPacked,'uint8');
blankMessage.data(1:numel(dataCasted)) = dataCasted;
blankMessage.data_SL_Info.CurrentLength = uint32(numel(dataCasted));

msg = blankMessage;

== matlab function point_cloud_filter_transform_node/For Iterator Subsystem/If Action Subsystem1/Affine ==
  data: out output; u input
function out = fcn(u)

tform = affine3d;
pt = pointCloud(u);
xyz = pctransform(pt,tform);
out = xyz.Location;

== matlab function point_cloud_filter_transform_node/For Iterator Subsystem/If Action Subsystem1/add_point_to_cloud/MATLAB Function ==
  data: cloud output size=[55000 3]; cloud input; pt input; idx input
function cloud = fcn(cloud,pt, idx)
cloud(idx,:) = pt;

== matlab function point_cloud_filter_transform_node/For Iterator Subsystem/If Action Subsystem1/add_point_to_cloud1/MATLAB Function ==
  data: Intensity input; j input; Intensity output size=55000; intensity input
function Intensity = fcn(Intensity, j, intensity)

Intensity(j,:) = intensity;
